simulink model "HarnessModel_BEVController"  (R2024b)
settings: Solver=daessc  StartTime=0.0  StopTime=2000  RelTol=1e-3  AbsTol=1e-3
PreLoadFcn:
  | HarnessSetup_BEVController
settings Model: Creator=isaacito  LastModifiedBy=ythvg
settings SolverCC: AutoScaleAbsTol=off  AlgebraicLoopSolver=TrustRegion
settings DataIOCC: DSMLogging=off
settings OptimizationCC: ReuseModelBlockBuffer=off
settings DebuggingCC: UnconnectedInputMsg=warning  UnconnectedOutputMsg=warning  UnconnectedLineMsg=warning
settings ModelReferenceCC: EnableRefExpFcnMdlSchedulingChecks=on
settings RTWCC: GPUComputeCapability=3.5  DLArmComputeVersion=19.05
settings SimscapeCC: SimscapeLogType=all  SimscapeLogSimulationStatistics=on  SimscapeLogLimitData=off

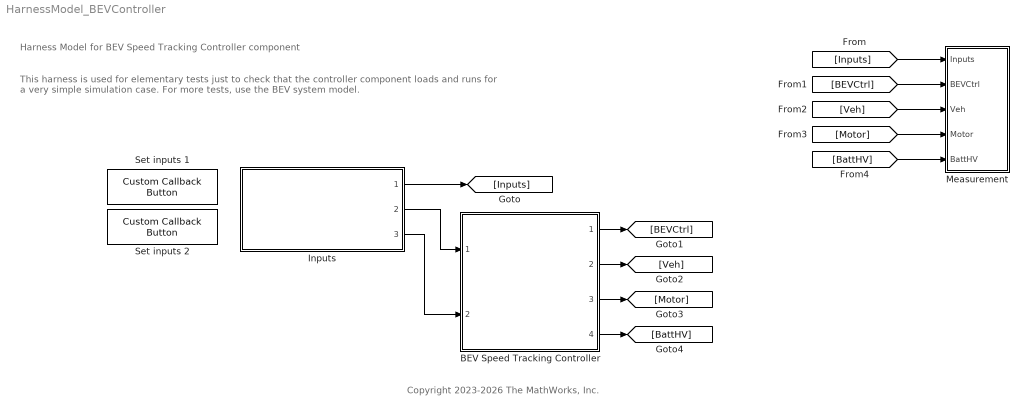
== system HarnessModel_BEVController ==
  note: This harness is used for elementary tests
      | just to check that the controller component loads and runs
      | for a very simple simulation case.
      | For more tests, use the BEV system model.
  note: Harness Model for BEV Speed Tracking Controller component
  note: Copyright 2023-2026 The MathWorks, Inc.
  BEV Speed Tracking Controller : Subsystem  ReferencedSubsystem=BEVController_Basic_refsub
      settings: OpenFcn=|
      | % Look under mask:
      | open_system(gcb, "force")
  Inputs : Subsystem  ReferencedSubsystem=Inputs_BEVController_Random_refsub
      settings: OpenFcn="open_system(gcb, \"force\")"
  Measurement : Subsystem
  Set inputs 1 : CustomCallbackButton  Configuration="{\"components\":[{\"name\":\"BackgroundImageComponent\",\"settings\":{\"image\":{\"size\":[0,0],\"src\":\"default\",\"srcOrientation\":\"Right\"},\"position\":[0,0,1,1]}},{\"name\":\"ButtonStateComponent\",\"settings\":{\"buttonType\":\"momentary\",\"clickFcn\":\"set_param(gcs + \\\"\\/Inputs\\\", ReferencedSubsystem=\\\"Inputs_BEVController_Simple_refsub\\\")\\nset_param(gcs, StopTime=\\\"600\\\")\",\"onValue\":1,\"position\":[0,0,1,1],\"pressDelay\":\"500\",\"pressFcn\":\"\",\"repeatInterval\":\"0\",\"states\":[{\"horizontalAlignment\":\"center\",\"image\":{\"position\":[0,0,1,1],\"size\":[1,1],\"src\":\"default\",\"srcOrientation\":\"Right\"},\"label\":{\"color\":[0.01176470588,0.01176470588,0.01176470588,1],\"icon\":{\"size\":[0,0],\"src\":\"default\",\"srcOrientation\":\"Right\"},\"iconOffset\":0,\"iconPlacement\":\"left\",\"opacity\":1,\"show\":true,\"text\":{\"content\":\"Simple\",\"font\":\"Helvetica\"}},\"labelOffset\":[0,0],\"verticalAlignment\":\"middle\"},{\"horizontalAlignment\":\"center\",\"image\":{\"position\":[0,0,1,1],\"size\":[1,1],\"src\":\"default\",\"srcOrientation\":\"Right\"},\"label\":{\"color\":[0.01176470588,0.01176470588,0.01176470588,1],\"icon\":{\"size\":[0,0],\"src\":\"default\",\"srcOrientation\":\"Right\"},\"iconOffset\":0,\"iconPlacement\":\"left\",\"opacity\":1,\"show\":true,\"text\":{\"content\":\"Simple\",\"font\":\"Helvetica\"}},\"labelOffset\":[0,0],\"verticalAlignment\":\"middle\"},{\"horizontalAlignment\":\"center\",\"image\":{\"position\":[0,0,1,1],\"size\":[1,1],\"src\":\"default\",\"srcOrientation\":\"Right\"},\"label\":{\"color\":[0.01176470588,0.01176470588,0.01176470588,1],\"icon\":{\"size\":[0,0],\"src\":\"default\",\"srcOrientation\":\"Right\"},\"iconOffset\":0,\"iconPlacement\":\"left\",\"opacity\":1,\"show\":true,\"text\":{\"content\":\"Simple\",\"font\":\"Helvetica\"}},\"labelOffset\":[0,0],\"verticalAlignment\":\"middle\"},{\"horizontalAlignment\":\"center\",\"image\":{\"position\":[0,0,1,1],\"size\":[1,1],\"src\":\"default\",\"srcOrientation\":\"Right\"},\"label\":{\"color\":[0.01176470588,0.01176470588,0.01176470588,1],\"icon\":{\"size\":[0,0],\"src\":\"default\",\"srcOrientation\":\"Right\"},\"iconOffset\":0,\"iconPlacement\":\"left\",\"opacity\":1,\"show\":true,\"text\":{\"content\":\"Simple\",\"font\":\"Helvetica\"}},\"labelOffset\":[0,0],\"verticalAlignment\":\"middle\"}]}},{\"name\":\"ForegroundImageComponent\",\"settings\":{\"image\":{\"size\":[0,0],\"src\":\"default\",\"srcOrientation\":\"Right\"},\"isForeground\":1,\"position\":[0,0,1,1]}}],\"derived\":{\"blockParameters\":{\"AutoActivate\":true,\"ButtonText\":\"Simple\",\"ButtonType\":\"Momentary\",\"ClickFcn\":\"set_param(gcs + \\\"\\/Inputs\\\", ReferencedSubsystem=\\\"Inputs_BEVController_Simple_refsub\\\")\\nset_param(gcs, StopTime=\\\"600\\\")\",\"OnValue\":1,\"PressDelay\":\"500\",\"PressFcn\":\"\",\"RepeatInterval\":\"0\",\"fixedAspectRatio\":\"off\"}},\"settings\":{\"BindingType\":\"standalone\",\"autoActivate\":true,\"backgroundColor\":[244,244,244,1],\"backgroundOffset\":0.2,\"backgroundOpacity\":1,\"fixedAspectRatio\":\"off\",\"foregroundColor\":[0.01176470588,0.01176470588,0.01176470588,1],\"migratedFromLegacy\":true,\"useBackgroundColor\":true,\"variant\":\"callback\",\"version\":\"R2024b\"},\"type\":\"Button\"}"  CustomBackgroundColor="{\"color\":[0.9568627451,0.9568627451,0.9568627451],\"show\":true}"
  Set inputs 2 : CustomCallbackButton  Configuration="{\"components\":[{\"name\":\"BackgroundImageComponent\",\"settings\":{\"image\":{\"size\":[0,0],\"src\":\"default\",\"srcOrientation\":\"Right\"},\"position\":[0,0,1,1]}},{\"name\":\"ButtonStateComponent\",\"settings\":{\"buttonType\":\"momentary\",\"clickFcn\":\"set_param(gcs + \\\"\\/Inputs\\\", ReferencedSubsystem=\\\"Inputs_BEVController_Random_refsub\\\")\\nset_param(gcs, StopTime=\\\"2000\\\")\",\"onValue\":1,\"position\":[0,0,1,1],\"pressDelay\":\"500\",\"pressFcn\":\"\",\"repeatInterval\":\"0\",\"states\":[{\"horizontalAlignment\":\"center\",\"image\":{\"position\":[0,0,1,1],\"size\":[1,1],\"src\":\"default\",\"srcOrientation\":\"Right\"},\"label\":{\"color\":[0.01176470588,0.01176470588,0.01176470588,1],\"icon\":{\"size\":[0,0],\"src\":\"default\",\"srcOrientation\":\"Right\"},\"iconOffset\":0,\"iconPlacement\":\"left\",\"opacity\":1,\"show\":true,\"text\":{\"content\":\"Random\",\"font\":\"Helvetica\"}},\"labelOffset\":[0,0],\"verticalAlignment\":\"middle\"},{\"horizontalAlignment\":\"center\",\"image\":{\"position\":[0,0,1,1],\"size\":[1,1],\"src\":\"default\",\"srcOrientation\":\"Right\"},\"label\":{\"color\":[0.01176470588,0.01176470588,0.01176470588,1],\"icon\":{\"size\":[0,0],\"src\":\"default\",\"srcOrientation\":\"Right\"},\"iconOffset\":0,\"iconPlacement\":\"left\",\"opacity\":1,\"show\":true,\"text\":{\"content\":\"Random\",\"font\":\"Helvetica\"}},\"labelOffset\":[0,0],\"verticalAlignment\":\"middle\"},{\"horizontalAlignment\":\"center\",\"image\":{\"position\":[0,0,1,1],\"size\":[1,1],\"src\":\"default\",\"srcOrientation\":\"Right\"},\"label\":{\"color\":[0.01176470588,0.01176470588,0.01176470588,1],\"icon\":{\"size\":[0,0],\"src\":\"default\",\"srcOrientation\":\"Right\"},\"iconOffset\":0,\"iconPlacement\":\"left\",\"opacity\":1,\"show\":true,\"text\":{\"content\":\"Random\",\"font\":\"Helvetica\"}},\"labelOffset\":[0,0],\"verticalAlignment\":\"middle\"},{\"horizontalAlignment\":\"center\",\"image\":{\"position\":[0,0,1,1],\"size\":[1,1],\"src\":\"default\",\"srcOrientation\":\"Right\"},\"label\":{\"color\":[0.01176470588,0.01176470588,0.01176470588,1],\"icon\":{\"size\":[0,0],\"src\":\"default\",\"srcOrientation\":\"Right\"},\"iconOffset\":0,\"iconPlacement\":\"left\",\"opacity\":1,\"show\":true,\"text\":{\"content\":\"Random\",\"font\":\"Helvetica\"}},\"labelOffset\":[0,0],\"verticalAlignment\":\"middle\"}]}},{\"name\":\"ForegroundImageComponent\",\"settings\":{\"image\":{\"size\":[0,0],\"src\":\"default\",\"srcOrientation\":\"Right\"},\"isForeground\":1,\"position\":[0,0,1,1]}}],\"derived\":{\"blockParameters\":{\"AutoActivate\":true,\"ButtonText\":\"Random\",\"ButtonType\":\"Momentary\",\"ClickFcn\":\"set_param(gcs + \\\"\\/Inputs\\\", ReferencedSubsystem=\\\"Inputs_BEVController_Random_refsub\\\")\\nset_param(gcs, StopTime=\\\"2000\\\")\",\"OnValue\":1,\"PressDelay\":\"500\",\"PressFcn\":\"\",\"RepeatInterval\":\"0\",\"fixedAspectRatio\":\"off\"}},\"settings\":{\"BindingType\":\"standalone\",\"autoActivate\":true,\"backgroundColor\":[244,244,244,1],\"backgroundOffset\":0.2,\"backgroundOpacity\":1,\"fixedAspectRatio\":\"off\",\"foregroundColor\":[0.01176470588,0.01176470588,0.01176470588,1],\"migratedFromLegacy\":true,\"useBackgroundColor\":true,\"variant\":\"callback\",\"version\":\"R2024b\"},\"type\":\"Button\"}"  CustomBackgroundColor="{\"color\":[0.9568627451,0.9568627451,0.9568627451],\"show\":true}"
  wires:
  Inputs/2 -> BEV Speed Tracking Controller/1
  Inputs/3 -> BEV Speed Tracking Controller/2
  Inputs/1 -> [Inputs]
  BEV Speed Tracking Controller/1 -> [BEVCtrl]
  BEV Speed Tracking Controller/2 -> [Veh]
  BEV Speed Tracking Controller/3 -> [Motor]
  BEV Speed Tracking Controller/4 -> [BattHV]
  [Inputs] -> Measurement/1(Inputs)
  [BEVCtrl] -> Measurement/2(BEVCtrl)
  [Veh] -> Measurement/3(Veh)
  [Motor] -> Measurement/4(Motor)
  [BattHV] -> Measurement/5(BattHV)

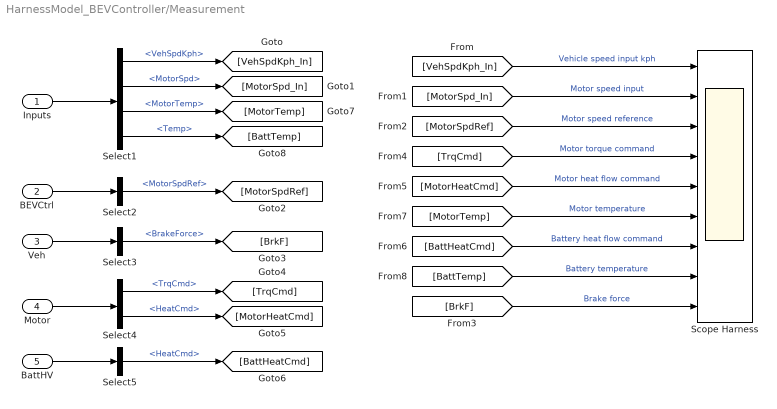
== system HarnessModel_BEVController/Measurement ==
  Inputs : Inport
  BEVCtrl : Inport  Port=2
  Veh : Inport  Port=3
  Motor : Inport  Port=4
  BattHV : Inport  Port=5
  Scope Harness : Scope  NumInputPorts=9
  Select1 : BusSelector  OutputSignals=VehicleSystem.Vehicle.VehSpdKph,VehicleSystem.Motor.MotorSpd,VehicleSystem.Motor.MotorTemp,VehicleSystem.Battery.Temp
  Select2 : BusSelector  OutputSignals=MotorSpdRef
  Select3 : BusSelector  OutputSignals=BrakeForce
  Select4 : BusSelector  OutputSignals=TrqCmd,HeatCmd
  Select5 : BusSelector  OutputSignals=HeatCmd
  wires:
  Inputs/1 -> Select1/1
  Select1/1 -> [VehSpdKph_In]  "<VehSpdKph>"
  Select1/2 -> [MotorSpd_In]  "<MotorSpd>"
  BEVCtrl/1 -> Select2/1
  Select2/1 -> [MotorSpdRef]  "<MotorSpdRef>"
  Veh/1 -> Select3/1
  Select3/1 -> [BrkF]  "<BrakeForce>"
  Motor/1 -> Select4/1
  Select4/1 -> [TrqCmd]  "<TrqCmd>"
  Select4/2 -> [MotorHeatCmd]  "<HeatCmd>"
  BattHV/1 -> Select5/1
  Select5/1 -> [BattHeatCmd]  "<HeatCmd>"
  [VehSpdKph_In] -> Scope Harness/1  "Vehicle speed input kph"
  [MotorSpd_In] -> Scope Harness/2  "Motor speed input"
  [MotorSpdRef] -> Scope Harness/3  "Motor speed reference"
  Select1/3 -> [MotorTemp]  "<MotorTemp>"
  Select1/4 -> [BattTemp]  "<Temp>"
  [TrqCmd] -> Scope Harness/4  "Motor torque command"
  [MotorHeatCmd] -> Scope Harness/5  "Motor heat flow command"
  [MotorTemp] -> Scope Harness/6  "Motor temperature"
  [BattHeatCmd] -> Scope Harness/7  "Battery heat flow command"
  [BattTemp] -> Scope Harness/8  "Battery temperature"
  [BrkF] -> Scope Harness/9  "Brake force"
